simulink model "lab_4"  (R2020b)
settings: Solver=VariableStepAuto  StartTime=0.0  StopTime=9  MaxStep=0.001  RelTol=1e-3
settings Model: Creator=Eugene  LastModifiedBy=Eugene

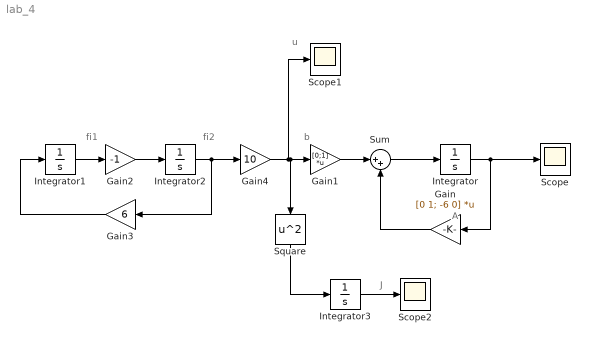
== system lab_4 ==
  note: u
  note: J
  note: fi1
  note: b
  note: A
  note: fi2
  Gain : Gain  Gain=[0 1; -6 0]  Multiplication=Matrix(K*u)
  Gain1 : Gain  Gain=[0;1]  Multiplication=Matrix(K*u)
  Gain2 : Gain  Gain=-1
  Gain3 : Gain  Gain=6
  Gain4 : Gain  Gain=10
  Integrator : Integrator  InitialCondition=[0;0]
  Integrator1 : Integrator  InitialCondition=-8.0071
  Integrator2 : Integrator  InitialCondition=-0.1790
  Integrator3 : Integrator
  Scope : Scope
  Scope1 : Scope
  Scope2 : Scope
  Square : Math  Operator=square  SaturateOnIntegerOverflow=on
  Sum : Sum  Inputs=|++
  wires:
  Integrator/1 -> Scope/1, Gain/1
  Sum/1 -> Integrator/1
  Gain1/1 -> Sum/1
  Gain/1 -> Sum/2
  Integrator2/1 -> Gain4/1, Gain3/1
  Integrator1/1 -> Gain2/1
  Gain2/1 -> Integrator2/1
  Gain3/1 -> Integrator1/1
  Gain4/1 -> Square/1, Gain1/1, Scope1/1
  Integrator3/1 -> Scope2/1
  Square/1 -> Integrator3/1
